simulink model "testemplanner_cs_old"  (R2020a)
settings: Solver=ode5  StartTime=0.0  StopTime=30  FixedStep=1/1000  RelTol=1e-3
PreLoadFcn:
  | mbxruntime.callbacks.PreLoadFcn(bdroot);
PostLoadFcn:
  | mbxruntime.callbacks.PostLoadFcn(bdroot);
InitFcn:
  | mbxruntime.callbacks.InitFcn(bdroot);
StartFcn:
  | mbxruntime.callbacks.StartFcn(bdroot);
StopFcn:
  | mbxruntime.callbacks.StopFcn(bdroot);
model workspace (MAT data in the model file):
  mbox_table : object (value not decoded)
  model_closed = 0
  sim_status = 0
values from neighbouring files (symbols this model uses):
  c_factor = 43.75    [emplanner_init.m]
  cf = -175016    [emplanner_init.m]
  cr = -130634    [emplanner_init.m]
  global_path_x = [-12.787 -11.7876177449 -10.7894946344 -9.79264775065 -8.79708287721 -7.80280164192 -6.80980414431 -5.81808992236 -4.82765830817 -3.83850855887 -2.85063990477 -1.86405156707 ... (3001 elements, 3001x1)]    [global_path.mat]
  global_path_y = [5.7602 5.7602 5.7602 5.7602 5.7602 5.7602 5.7602 5.7602 5.7602 5.7602 5.7602 5.7602 ... (3001 elements, 3001x1)]    [global_path.mat]
  KD_PID_distance = 0.0    (= 0)    [emplanner_init.m]
  KD_PID_speed = 0    [emplanner_init.m]
  KI_PID_distance = 0.0    (= 0)    [emplanner_init.m]
  KI_PID_speed = 0    [emplanner_init.m]
  KP_PID_distance = 0.5    [emplanner_init.m]
  KP_PID_speed = 1.8    [emplanner_init.m]
  la = 1.265    [emplanner_init.m]
  lb = 2.947-1.265    (= 1.682)    [emplanner_init.m]
  LQR_K1 = k(:,1)'    [emplanner_init.m]
  LQR_K2 = k(:,2)'    [emplanner_init.m]
  LQR_K3 = k(:,3)'    [emplanner_init.m]
  LQR_K4 = k(:,4)'    [emplanner_init.m]
  m = 2020    [emplanner_init.m]
  rack_displacement = [-39.14 , -37.2 , -35.29 , -33.43 , -31.6 , -29.81 , -28.06 , -26.34 , -24.66 ,      -23.01 , -21.38 , -19.79 , -18.23 , -16.69 , -15.18 , -13.7 , -12.23 , -10.8 , -9.38 , -7.98 ,     -6.61 , -5.25 , -3.91 , -2.59 , -1.29 , 0 , 1.27 , 2.54 , 3.78 , 5.02 , 6.24 , 7.46 , 8.66 ,      9.86 , 11.05 , 12.24 , 13.41 , 14.59 , 15.76 , 16.92 , 18.09 , 19.25 , 20.42 , 21.59 , 22.76 ,      23.93 , 25.11 , 26 ...(+26 chars)    [emplanner_init.m]
  right_wheel_ground = [-70 ,-67.2 , -64.4 , -61.6 , -58.8 , -56 , -53.2 , -50.4 , -47.6 , -44.8 , -42 ,      -39.2 , -36.4 , -33.6 , -30.8 , -28 , -25.2 , -22.4 , -19.6 , -16.8 , -14 , -11.2 , -8.4 , -5.6 ,      -2.8 , 0 , 2.8 , 5.6 , 8.4 , 11.2 , 14 , 16.8 , 19.6 , 22.4 , 25.2 , 28 , 30.8 , 33.6 , 36.4 ,      39.2 , 42 , 44.8 , 47.6 , 50.4 , 53.2 , 56 , 58.8 , 61.6 , 64.4 , 67.2 , 70 ]    [emplanner_init.m]
  vx_break_point = zeros(1,5000)    [emplanner_init.m]
undefined symbols (not defined in the file or in its folder): aubr, DiscIntNeverNeededParam, tablebr, vubr, warningInitialVelocity, x0
libraries: PreScanSimulinkLibrary x39, simulink x19, simulink_extras x11, Solver_SF x1
(part 12 of 17)

== matlab function testemplanner_cs_old/Audi_A8_Sedan_1/decision&planning module/EM Planner/path decision task1/path decision with dynamic planning(dp) ==
  data: obs_s_set input; dp_path_s output; obs_l_set input; plan_start_s input; plan_start_l input; plan_start_dl input; plan_start_dll input; w_cost_collision input; w_cost_smooth_dl input; w_cost_smooth_ddl input; w_cost_smooth_dddl input; w_cost_ref input; row input; col input; sample_s input; sample_l input; dp_path_l output
function [dp_path_s,dp_path_l] = fcn(obs_s_set,obs_l_set,plan_start_s,plan_start_l,plan_start_dl,...
    plan_start_dll,w_cost_collision,w_cost_smooth_dl,w_cost_smooth_ddl,w_cost_smooth_dddl,w_cost_ref,row,col,sample_s,sample_l)
%该函数为路径决策算法动态规划的主函数
% 输入：obs s l set 筛选后的障碍物sl信息
%       plan_start s l dl ddl 规划起点信息
%       w_cost_obs,w_cost_smooth_dl,w_cost_smooth_ddl,w_cost_smooth_dddl,w_cost_ref动态规划代价权重
%       row col 动态规划采样点的行数和列数(row必须是奇数，col必须是6)
%       sample_s,sample_l 采样的s l 长度
% 输出：dp_path_l,dp_path_s 动态规划的路径sl,此路径不包含规划起点  

%动态规划最优的数据结构是结构体矩阵，但是simulink不支持结构体矩阵，所以动态规划算法写的相对难以理解

%声明二维矩阵变量node_cost，node_cost(i,j)表示从起点出发，到行i列j节点的最小代价为node_cost(i,j)
node_cost = ones(row,col)*inf;%初始化为无穷大

%声明二维矩阵变量pre_node_index pre_node_index(i,j)表示从起点到行i列j的节点的最优路径中前一个节点的行号为
%pre_node_index(i,j)
%例：比如一条最优路径为 起点 -> node(1,1) -> node(2,2) -> node(3,3)
%则pre_node_index(3,3) = 2 (最优路径的前一个节点是node(2,2) 取它的行号）
%  pre_node_index(2,2) = 1 (最优路径的前一个节点是node(1,1) 取它的行号）
%  pre_node_index(1,1) = 0 (起点的行号默认是0)

% 其实pre_node_index就是当找到最小代价的路径后从终点到起点反向选择出最优路径的
%如果用结构体矩阵完全没有必要弄得这么麻烦，但是simulink不支持
pre_node_index = zeros(row,col);%初始化，所有节点的上个最优节点的行号都是0，也就是起点

%先计算从起点到第一列的cost
for i = 1:row
    node_cost(i,1) = CalcStartCost(plan_start_s,plan_start_l,plan_start_dl,...
    plan_start_dll,i,sample_s,sample_l,w_cost_collision,w_cost_smooth_dl,...
    w_cost_smooth_ddl,w_cost_smooth_dddl,w_cost_ref,obs_s_set,obs_l_set,row);
end
% 动态规划主函数，从第二列开始
for j = 2:col
    for i = 1:row
        %计算当前node(i,j)的s l
        cur_node_s = plan_start_s + j * sample_s;
        cur_node_l = ((row + 1)/2 - i) * sample_l;
        %遍历前一列的节点
        for k = 1:row
            %计算前一列节点的s l
            pre_node_s = plan_start_s + (j - 1) * sample_s;
            pre_node_l = ((row + 1)/2 - k) * sample_l;
            cost_neighbour = CalcNeighbourCost(pre_node_s,pre_node_l,cur_node_s,cur_node_l,w_cost_collision,...
    w_cost_smooth_dl,w_cost_smooth_ddl,w_cost_smooth_dddl,w_cost_ref,obs_s_set,obs_l_set);
            %起点到上一个节点的最小代价为node_cost(k,j-1)
            pre_min_cost = node_cost(k,j-1);
            %起点到node_cost(i,j)的最小代价 为node_cost(k,j-1)
            %再加上node(k,j-1)到node(i,j)的代价 (k = 1,2,3,4...row) 中最小的
            cost_temp = pre_min_cost + cost_neighbour;
            if cost_temp < node_cost(i,j)
                node_cost(i,j) = cost_temp;
                %把最优路径上一列节点的行号记录下来
                pre_node_index(i,j) = k;
            end
        end      
    end
end
%找到node_cost最后一列中，cost最小的，记代价最小的行号为index
index = 0;
min_cost = inf;
for i = 1:row
    if node_cost(i,end) < min_cost
        min_cost = node_cost(i,end);
        index = i;
    end
end
%动态规划最优路径初始化
dp_node_list_row = zeros(col,1);
%从后往前逆推
cur_index = index;
for i = 1:col
    %记录cur_index前面节点的行号
    pre_index = pre_node_index(cur_index,end - i + 1);
    %把cur_index放到dp_node_list_row对应的位置
    dp_node_list_row(col - i + 1) = cur_index;
    %再把pre_index 赋给 cur_index 进行下一步递推
    cur_index = pre_index;
end
% 输出初始化，由于事先不知道横纵向的采样列数，因此需要做缓冲
dp_path_s = ones(15,1)*-1;
dp_path_l = ones(15,1)*-1;
for i = 1:col
    dp_path_s(i) = plan_start_s + i * sample_s;
    dp_path_l(i) = ((row + 1) / 2 - dp_node_list_row(i)) * sample_l;
end








end
function cost = CalcNeighbourCost(pre_node_s,pre_node_l,cur_node_s,cur_node_l,w_cost_collision,...
    w_cost_smooth_dl,w_cost_smooth_ddl,w_cost_smooth_dddl,w_cost_ref,obs_s_set,obs_l_set)
% 该函数将计算相邻两个节点之间的cost
  
    start_l = pre_node_l;
    start_dl = 0;
    start_ddl = 0;
    end_l = cur_node_l;
    end_dl = 0;
    end_ddl = 0;
    start_s = pre_node_s;
    end_s = cur_node_s;
    coeff = CalcQuinticCoeffient(start_l,start_dl,start_ddl,end_l,end_dl,end_ddl,start_s,end_s);
    a0 = coeff(1);
    a1 = coeff(2);
    a2 = coeff(3);
    a3 = coeff(4);
    a4 = coeff(5);
    a5 = coeff(6);
    % 取10个点计算cost
    ds = zeros(10,1);
    l = zeros(10,1);
    dl = zeros(10,1);
    ddl = zeros(10,1);
    dddl = zeros(10,1);
    for i = 1:10
        ds(i) = start_s + (i-1)*(end_s - start_s)/10;
    end
    l = a0 * ones(10,1) + a1 * ds + a2 * ds.^2 + a3 * ds.^3 + a4 * ds.^4 + a5 * ds.^5;
    dl = a1 * ones(10,1) + 2 * a2 * ds + 3 * a3 * ds.^2 + 4 * a4 * ds.^3 + 5 * a5 * ds.^4;
    ddl = 2 * a2 * ones(10,1) + 6 * a3 * ds + 12 * a4 * ds.^2 + 20 * a5 * ds.^3;
    dddl = 6 * ones(10,1) * a3 + 24 * a4 * ds + 60 * a5 * ds.^2;
    cost_smooth = w_cost_smooth_dl * (dl' * dl) + w_cost_smooth_ddl * (ddl' * ddl) + w_cost_smooth_dddl * (dddl' * dddl);
    for i = 1:length(ddl)
        if abs(ddl(i))> 0.5 || abs(atan(dl(i))) > 0.4*pi
            cost_smooth = cost_smooth + 1e7;
            break;
        end
    end
    cost_ref = w_cost_ref * (l' * l);
    cost_collision = 0;
    for i = 1:length(obs_s_set)
        if isnan(obs_s_set(i))
            break;
        end
        dlon = ones(10,1) * obs_s_set(i) - ds;
        dlat = ones(10,1) * obs_l_set(i) - l;
        %这里做了非常简化的质点模型，认为障碍物就是一个点
        square_d = dlon.^2 + dlat.^2;
        cost_collision_once = CalcObsCost(w_cost_collision,square_d);
        cost_collision = cost_collision + cost_collision_once;
        % 判断障碍物的左右
        v1 = [ds(end);l(end)] - [ds(1);l(1)];
        v2 = [obs_s_set(i);obs_l_set(i)] - [ds(1);l(1)];
        flag = v1(1)*v2(2) - v1(2)*v2(1);
        if flag < 0 && cost_collision > 0
            cost_collision = cost_collision - 1000;
        end
    end
    
    cost = cost_collision + cost_smooth + cost_ref;


end


function cost = CalcStartCost(begin_s,begin_l,begin_dl,begin_ddl,cur_node_row,sample_s,sample_l,w_cost_collision,...
    w_cost_smooth_dl,w_cost_smooth_ddl,w_cost_smooth_dddl,w_cost_ref,obs_s_set,obs_l_set,row)
    %该函数将计算起点到第一层的cost
    start_l = begin_l;
    start_dl = begin_dl;
    start_ddl = begin_ddl;
    %  . . .
    %  . . . row = 3 中间的行号 = (row + 1) /2 = 2
    %  . . .
    end_l = ((row + 1)/2 - cur_node_row)*sample_l;
    end_dl = 0;
    end_ddl = 0;
    start_s = begin_s;
    end_s = begin_s + sample_s;
    coeff = CalcQuinticCoeffient(start_l,start_dl,start_ddl,end_l,end_dl,end_ddl,start_s,end_s);
    a0 = coeff(1);
    a1 = coeff(2);
    a2 = coeff(3);
    a3 = coeff(4);
    a4 = coeff(5);
    a5 = coeff(6);
    % 取10个点计算cost
    ds = zeros(10,1);
    l = zeros(10,1);
    dl = zeros(10,1);
    ddl = zeros(10,1);
    dddl = zeros(10,1);
    for i = 1:10
        ds(i) = start_s + (i-1)*sample_s/10;
    end
    l = a0 * ones(10,1) + a1 * ds + a2 * ds.^2 + a3 * ds.^3 + a4 * ds.^4 + a5 * ds.^5;
    dl = a1 * ones(10,1) + 2 * a2 * ds + 3 * a3 * ds.^2 + 4 * a4 * ds.^3 + 5 * a5 * ds.^4;
    ddl = 2 * a2 * ones(10,1) + 6 * a3 * ds + 12 * a4 * ds.^2 + 20 * a5 * ds.^3;
    dddl = 6 * ones(10,1) * a3 + 24 * a4 * ds + 60 * a5 * ds.^2;
    cost_smooth = w_cost_smooth_dl * (dl' * dl) + w_cost_smooth_ddl * (ddl' * ddl) + w_cost_smooth_dddl * (dddl' * dddl);
    for i = 1:length(dl)
        if abs(ddl(i))> 0.5 || abs(atan(dl(i))) > 0.4*pi
            cost_smooth = cost_smooth + 1e7;
            break;
        end
    end
    cost_ref = w_cost_ref * (l' * l);
    cost_collision = 0;
    for i = 1:length(obs_s_set)
        if isnan(obs_s_set(i))
            break;
        end
        dlon = ones(10,1) * obs_s_set(i) - ds;
        dlat = ones(10,1) * obs_l_set(i) - l;
        %这里做了非常简化的质点模型，认为障碍物就是一个点
        square_d = dlon.^2 + dlat.^2;
        cost_collision_once = CalcObsCost(w_cost_collision,square_d);
        cost_collision = cost_collision + cost_collision_once;
        % 判断障碍物的左右
        v1 = [ds(end);l(end)] - [ds(1);l(1)];
        v2 = [obs_s_set(i);obs_l_set(i)] - [ds(1);l(1)];
        flag = v1(1)*v2(2) - v1(2)*v2(1);
        if flag < 0 && cost_collision > 0
            cost_collision = cost_collision - 1000;
        end
    end
    
    cost = cost_collision + cost_smooth + cost_ref;
        
end

function obs_cost = CalcObsCost(w_cost_collision,square_d)
%该函数将计算障碍物的距离代价
% 暂定超过4米的cost为0 在4到3米的cost为1000/squard_d,在小于3米的cost为w_cost_collision
%   cost = 0;
%   for i = 1:length(square_d)
%       if (square_d(i) < 16 && square_d(i) > 9) 
%           cost = cost + 500/square_d(i);
%       elseif (square_d(i) <= 9)
%           cost = cost + w_cost_collision;
%       end
%   end
%   obs_cost = cost;
min_d = inf;
for i = 1:length(square_d)
    min_d = min(min_d,square_d(i));
end
    obs_cost = w_cost_collision * 10^(-min_d/3);
end

function coeff = CalcQuinticCoeffient(start_l,start_dl,start_ddl,end_l,end_dl,end_ddl,start_s,end_s)
    % l = a0 + a1*s + a2*s^2 + a3*s^3 + a4*s^4 + a5*s^5
    % l' = a1 + 2 * a2 * s + 3 * a3 * s^2 + 4 * a4 * s^3 + 5 * a5 * s^4
    % l'' = 2 * a2 + 6 * a3 * s + 12 * a4 * s^2 + 20 * a5 * s^3
    start_s2 = start_s * start_s;
    start_s3 = start_s2 * start_s;
    start_s4 = start_s3 * start_s;
    start_s5 = start_s4 * start_s;
    end_s2 = end_s * end_s;
    end_s3 = end_s2 * end_s;
    end_s4 = end_s3 * end_s;
    end_s5 = end_s4 * end_s;
    A = [1,start_s, start_s2,     start_s3,     start_s4,      start_s5;
         0 1,       2 * start_s,  3 * start_s2, 4 * start_s3,  5 * start_s4;
         0 0,       2,            6 * start_s,  12 * start_s2, 20 * start_s3;
         1,end_s, end_s2,     end_s3,     end_s4,      end_s5;
         0,1,     2 * end_s,  3 * end_s2, 4 * end_s3,  5 * end_s4;
         0,0,     2,          6 * end_s,  12 * end_s2, 20 * end_s3;];
    B = [start_l;
         start_dl;
         start_ddl;
         end_l;
         end_dl;
         end_ddl;];
     coeff = A \ B;
    
end

== matlab function testemplanner_cs_old/Audi_A8_Sedan_1/decision&planning module/referenceline provider/MATLAB Function4 ==
  data: referenceline_x_init input; referenceline_x output; referenceline_y_init input; w_cost_smooth input; w_cost_length input; w_cost_ref input; x_lb input; x_ub input; y_lb input; y_ub input; referenceline_y output
function [referenceline_x,referenceline_y] = ...
    fcn(referenceline_x_init,referenceline_y_init,w_cost_smooth,w_cost_length,w_cost_ref,x_lb,x_ub,y_lb,y_ub)
%该函数用于平滑referenceline
%使用二次规划
% 0.5x'Hx + f'x = min
% lb < x < ub
% 输入： referenceline_x_init,referenceline_y_init未平滑的参考线
%       w_cost_smooth,w_cost_length,w_cost_ref 平滑代价、紧凑代价、几何相似代价权重系数
%       x_lb,x_ub,y_lb,y_ub 允许x，y变化的上下界
%输出：referenceline_x,referenceline_y 平滑后的参考线

% 在这里为了简化，不使用参考线拼接算法
% 计算量问题通过调度解决，规划周期为100ms，只要在100ms内计算完就可以
% 如果到最后计算速度成问题再优化，目前暂时不适用拼接

% simulink无法直接使用自带的二次规划函数，需要从外部引入

coder.extrinsic("quadprog")
% 二次规划形式 （详见第二章第二节上）
% H1 = w_cost_smooth*(A1'*A1) + w_cost_length*(A2'*A2) + w_cost_ref*(A3'*A3)
% f = -2 * w_cost_ref * referenceline_init
% x'H1x + f'x = 0.5 * x'(2H1) * x + f'x
% A1 = [1  0 -2  0  1  0
%       0  1  0 -2  0  1
%             1  0 -2  0  1  0
%             0  1  0 -2  0  1
%                   ...............
% A2 = [1  0 -1  0
%      0  1  0 -1
%            1  0 -1  0
%            0  1  0 -1
%                  ...........
% A3 为单位矩阵
%设置求解矩阵规模，因为参考线初始点一共181个，每个点有两个坐标，所以求解矩阵规模是362个
n = 181;
%referenceline初始化
referenceline_x = zeros(n,1);
referenceline_y = zeros(n,1);

A1 = zeros(2 * n - 4, 2 * n);
A2 = zeros(2 * n - 2, 2 * n);
A3 = eye(2 * n, 2 * n);
f = zeros(2 * n, 1);
lb = zeros(2 * n, 1);
ub = zeros(2 * n, 1);
persistent is_first_run;
persistent pre_result_x;
persistent pre_result_y;
persistent pre_referenceline_x_init;
persistent pre_referenceline_y_init;

if isempty(is_first_run)
    is_first_run = 0;
    for i = 1 : n
        f(2 * i - 1) = referenceline_x_init(i);
        f(2 * i) = referenceline_y_init(i);
        lb(2 * i - 1) = f(2 * i - 1) + x_lb;
        ub(2 * i - 1) = f(2 * i - 1) + x_ub;
        lb(2 * i) = f(2 * i) + y_lb;
        ub(2 * i) = f(2 * i) + y_ub;
    end

    for j = 1 : 2 : 2 * n - 5   %A1维度2n-4 * 2n
        A1(j , j) = 1;
        A1(j , j + 2) = -2;
        A1(j , j + 4) = 1;
        A1(j + 1, j + 1) = 1;
        A1(j + 1, j + 3) = -2;
        A1(j + 1, j + 5) = 1;
    end

    for k = 1 : 2: 2 * n - 3
        A2(k, k) = 1;
        A2(k, k + 2) = -1;
        A2(k + 1, k + 1) = 1;
        A2(k + 1, k + 3) = -1;
    end

    H1 = w_cost_smooth * (A1'*A1) + w_cost_length * (A2'*A2) + w_cost_ref * (A3);
    H = 2 * H1;
    %用 referenceline 的初值作为二次规划的迭代起点
    X0 = f;
    f = -2 * w_cost_ref * f;
    %二次规划求解
    X = quadprog(H,f,[],[],[],[],lb,ub,X0);
    %将结果输出到referenceline中
    for i = 1 : n
       referenceline_x(i) = X(2 * i - 1);
       referenceline_y(i) = X(2 * i);
    end
    pre_result_x = referenceline_x;
    pre_result_y = referenceline_y;
    pre_referenceline_x_init = referenceline_x_init;
    pre_referenceline_y_init = referenceline_y_init;
else
    %起点相同，可以认为本周期和上周期的referenceline_init 一模一样，就直接复用上个周期的结果
    if pre_referenceline_x_init(1) == referenceline_x_init(1) && ...
            pre_referenceline_y_init(1) == referenceline_y_init(1)
        referenceline_x = pre_result_x;
        referenceline_y = pre_result_y;
    else
        %起点不同。重复第一次运行的逻辑
        for i = 1 : n
            f(2 * i - 1) = referenceline_x_init(i);
            f(2 * i) = referenceline_y_init(i);
            lb(2 * i - 1) = f(2 * i - 1) + x_lb;
            ub(2 * i - 1) = f(2 * i - 1) + x_ub;
            lb(2 * i) = f(2 * i) + y_lb;
            ub(2 * i) = f(2 * i) + y_ub;
        end

        for j = 1 : 2: 2 * n - 5
            A1(i , i) = 1;
            A1(i , i + 2) = -2;
            A1(i , i + 4) = 1;
            A1(i + 1, i + 1) = 1;
            A1(i + 1, i + 3) = -2;
            A1(i + 1, i + 5) = 1;
        end

        for k = 1 : 2: 2 * n - 3
            A2(i, i) = 1;
            A2(i, i + 2) = -1;
            A2(i + 1, i + 1) = 1;
            A2(i + 1, i + 3) = -1;
        end

        H1 = w_cost_smooth * (A1'*A1) + w_cost_length * (A2'*A2) + w_cost_ref * A3;
        H = 2 * H1;
        %用 referenceline 的初值作为二次规划的迭代起点
        X0 = f;
        f = -2 * w_cost_ref * f;
        %二次规划求解
        X = quadprog(H,f,[],[],[],[],lb,ub,X0);
        %将结果输出到referenceline中
        for i = 1 : n
            referenceline_x(i) = X(2 * i - 1);
            referenceline_y(i) = X(2 * i);
        end
        pre_result_x = referenceline_x;
        pre_result_y = referenceline_y;
        pre_referenceline_x_init = referenceline_x_init;
        pre_referenceline_y_init = referenceline_y_init;        
    end
end

== matlab function testemplanner_cs_old/Audi_A8_Sedan_1/decision&planning module/EM Planner/path planning task1/MATLAB Function ==
  data: qp_path_s input; qp_path_s_final output; qp_path_l input; qp_path_dl input; qp_path_ddl input; qp_path_l_final output; qp_path_dl_final output; qp_path_ddl_final output
function [qp_path_s_final,qp_path_l_final, qp_path_dl_final,qp_path_ddl_final] = fcn(qp_path_s,qp_path_l,qp_path_dl,qp_path_ddl)
% 该函数将增密qp_path
n_init = 20;
% 增密的点的个数
n = 501;
% 输出初始化
qp_path_s_final = zeros(n,1);
qp_path_l_final = zeros(n,1);
qp_path_dl_final = zeros(n,1);
qp_path_ddl_final = zeros(n,1);
ds = (qp_path_s(end) - qp_path_s(1))/(n-1);
index = 1;
for i = 1:n
    x = qp_path_s(1) + (i-1) * ds;
    qp_path_s_final(i) = x;
    while x >= qp_path_s(index)
        index = index + 1;
        if index == n_init
            break;
        end
    end
    % while 循环退出的条件是x<qp_path_s(index)，所以x对应的前一个s的编号是index-1 后一个编号是index
    pre = index - 1;
    cur = index;
    % 计算前一个点的l l' l'' ds 和后一个点的 l''
    delta_s = x - qp_path_s(pre);
    l_pre = qp_path_l(pre);
    dl_pre = qp_path_dl(pre);
    ddl_pre = qp_path_ddl(pre);
    ddl_cur = qp_path_ddl(cur);
    % 分段加加速度优化 
    qp_path_l_final(i) = l_pre + dl_pre * delta_s + (1/3)* ddl_pre * delta_s^2 + (1/6) * ddl_cur * delta_s^2;
    qp_path_dl_final(i) = dl_pre + 0.5 * ddl_pre * delta_s + 0.5 * ddl_cur * delta_s;
    qp_path_ddl_final(i) = ddl_pre + (ddl_cur - ddl_pre) * delta_s/(qp_path_s(cur) - qp_path_s(pre));
    %  因为此时x的后一个编号是index 必有x < qp_path_s(index),在下一个循环中x = x + ds 也未必大于
    %  qp_path_s(index)，这样就进入不了while循环，所以index 要回退一位
    index = index - 1;   
end

== matlab function testemplanner_cs_old/Audi_A8_Sedan_1/decision&planning module/EM Planner/path planning task1/generate convex space ==
  data: dp_path_s input; l_min output; dp_path_l input; static_obs_s_set input; static_obs_l_set input; static_obs_length input; static_obs_width input; l_max output
function [l_min,l_max] = fcn(dp_path_s,dp_path_l,static_obs_s_set,static_obs_l_set,static_obs_length,static_obs_width)
    % 该函数将输出每个离散的dp_path_s所对应的l的边界lmin lmax (本质上是质点的凸空间)
    % 输入 动态规划曲线 dp_path_s,dp_path_l
    %      障碍物中心的s l 坐标 static_obs_s,static_obs_l
    %      障碍物的长宽 static_obs_length,static_obs_width 
    % 输出 l_min lmax l 的上下界

    % 输出初始化
    l_min = ones(60,1) * -8;
    l_max = ones(60,1) * 8;
    % 对每个障碍物做遍历
    for i = 1:length(static_obs_s_set)
        if isnan(static_obs_s_set(i))
            break;
        end
        % 计算障碍物的头部和尾部的s
        obs_s_min = static_obs_s_set(i) - static_obs_length/2;
        obs_s_max = static_obs_s_set(i) + static_obs_length/2;
        % 找到dp_path_s 中，与s_head s_end最近的s的编号
        start_index = FindNearIndex(dp_path_s,obs_s_min);
        end_index = FindNearIndex(dp_path_s,obs_s_max);
        path_l = (dp_path_l(start_index) + dp_path_l(end_index))/2;
        if start_index == 1 && end_index == 1
            continue;
        end
        if path_l > static_obs_l_set(i)
            % 意味着决策为向左绕过障碍物
            for j = start_index:end_index
                % l_min(j) 为所有决策为向左绕过障碍物的l边界的最大值
                l_min(j) = max(l_min(j) , static_obs_l_set(i) + static_obs_width/2);
            end
        else
            % 意味着决策为向右绕过障碍物
            for j = start_index:end_index
                % l_max(j) 为所有决策为向右绕过障碍物的l边界的最小值
                l_max(j) = min(l_max(j) , static_obs_l_set(i) - static_obs_width/2);
            end
        end       
    end
end

function y = FindNearIndex(dp_path_s,obs_s)
    % 该函数将找到dp_path_s的所有点中，距离obs_s最近的点的编号
    % 这里要注意obs_s 是在完整的reference line上投影所得到的坐标，所以obs_s可能是负值，也可能会超过dp_path_s最远的长度
    if dp_path_s(1) >= obs_s
        %障碍物在后面
        y = 1;
        return;
    elseif dp_path_s(end) <= obs_s
        y = 60;
        return;
    else
        index = 1;
        while dp_path_s(index) < obs_s
            index = index + 1;
        end
        % 循环退出的条件是dp_path_s(index) >= obs_s 判断一下index 和 index-1哪个离的近
        if dp_path_s(index) - obs_s > obs_s - dp_path_s(index - 1)
            y = index - 1;
        else
            y = index;
        end
    end
end

== matlab function testemplanner_cs_old/Audi_A8_Sedan_1/decision&planning module/EM Planner/path planning task1/path planning with quadratic programming (qp) ==
  data: qp_path_s output; l_min input; qp_path_l output; l_max input; w_cost_l input; w_cost_dl input; w_cost_ddl input; w_cost_dddl input; w_cost_centre input; w_cost_end_l input; w_cost_end_dl input; w_cost_end_ddl input; host_d1 input; host_d2 input; host_w input; plan_start_s input; plan_start_l input; plan_start_dl input; plan_start_ddl input; qp_path_dl output; qp_path_ddl output; delta_dl_max input; delta_ddl_max input
function [qp_path_s,qp_path_l,qp_path_dl,qp_path_ddl] = ...
fcn(l_min,l_max,w_cost_l,w_cost_dl,w_cost_ddl,w_cost_dddl,w_cost_centre,w_cost_end_l,w_cost_end_dl,w_cost_end_ddl,...
    host_d1,host_d2,host_w,...
    plan_start_s,plan_start_l,plan_start_dl,plan_start_ddl,...
    delta_dl_max,delta_ddl_max)
% 路径二次规划
% 0.5*x'Hx + f'*x = min
% subject to A*x <= b
%            Aeq*x = beq
%            lb <= x <= ub;
% 输入：l_min l_max 点的凸空间
%       w_cost_l 参考线代价
%       w_cost_dl ddl dddl 光滑性代价
%       w_cost_centre 凸空间中央代价
%       w_cost_end_l dl dd1 终点的状态代价 (希望path的终点状态为(0,0,0))
%       host_d1,d2 host质心到前后轴的距离
%       host_w host的宽度
%       plan_start_l,dl,ddl 规划起点
% 输出 qp_path_l dl ddl 二次规划输出的曲线
coder.extrinsic("quadprog");
% 待优化的变量的数量
n = 20;

% 输出初始化
qp_path_l = zeros(n,1);
qp_path_dl = zeros(n,1);
qp_path_ddl = zeros(n,1);
qp_path_s = zeros(n,1);

% H_L H_DL H_DDL H_DDDL Aeq beq A b 初始化
H_L = zeros(3*n, 3*n);
H_DL = zeros(3*n, 3*n);
H_DDL = zeros(3*n, 3*n);
H_DDDL = zeros(n-1, 3*n);
H_CENTRE = zeros(3*n, 3*n);
H_L_END = zeros(3*n, 3*n);
H_DL_END = zeros(3*n, 3*n);
H_DDL_END = zeros(3*n, 3*n);
Aeq = zeros(2*n-2, 3*n);
beq = zeros(2*n-2, 1);
A = zeros(8*n, 3*n);
b = zeros(8*n, 1);
% 更新：加入 dl(i+1) - dl(i) ddl(i+1) - ddl(i) 的约束
A_dl_minus = zeros(n - 1,3*n);
b_dl_minus = zeros(n - 1,1);
A_ddl_minus = zeros(n - 1,3*n);
b_ddl_minus = zeros(n - 1,1);
for i = 1:n-1
    row = i;
    col = 3*i - 2;
    A_dl_minus(row,col:col+5) = [0 -1 0 0 1 0];
    b_dl_minus(row) = delta_dl_max;
    A_ddl_minus(row,col:col+5) = [0 0 -1 0 0 1];
    b_ddl_minus(row) = delta_ddl_max;
end
% -max < a*x < max => ax < max && -ax < -(-max)
A_minus = [A_dl_minus;
          -A_dl_minus;
           A_ddl_minus;
          -A_ddl_minus];
b_minus = [b_dl_minus;
           b_dl_minus;
          b_ddl_minus;
          b_ddl_minus]; 

%  期望的终点状态
end_l_desire = 0;
end_dl_desire = 0;
end_ddl_desire = 0;

% Aeq_sub
ds = 3;%纵向间隔
for i = 1:n
    qp_path_s(i) = plan_start_s + (i-1)*ds;
end

Aeq_sub = [1 ds ds^2/3 -1 0 ds^2/6;
           0 1  ds/2   0 -1 ds/2];
% A_sub;
d1 = host_d1;
d2 = host_d2;
w = host_w;
A_sub = [1  d1 0;
         1  d1 0;
         1 -d2 0;
         1 -d2 0;
        -1 -d1 0;
        -1 -d1 0;
        -1  d2 0;
        -1  d2 0];
% 生成Aeq
for i = 1:n-1
    % 计算分块矩阵左上角的行和列
    row = 2*i - 1;
    col = 3*i - 2;
    Aeq(row:row + 1,col:col + 5) = Aeq_sub;
end
% 生成A
for i = 2:n
    row = 8*i - 7;
    col = 3*i - 2;
    A(row:row + 7,col:col + 2) = A_sub;
end

% 视频里用的找(s(i) - d2,s(i) + d1)的方法过于保守，在这里舍弃掉
% 只要找到四个角点所对应的l_min l_max 即可
% 。。。。。。。。。。。。。。
%    [    .   ]<- 
%    [        ]
% 。。。。。。。。。。。。。
front_index = ceil(d1/ds);
back_index = ceil(d2/ds); % ceil向上取整 ceil(3) = 3 ceil(3.1) = 4
% 生成b
for i = 2:n
    % 左前 右前的index = min(i + front_index,60)
    % 左后 右后的index = max(i - back_index,1)
    % l_min l_max 都是60个点
    index1 = min(3*i - 2 + front_index,n);
    index2 = max(3*i - 2 - back_index,1);
    b(8*i - 7:8*i,1) = [l_max(index1) - w/2;
                        l_max(index1) + w/2;
                        l_max(index2) - w/2;
                        l_max(index2) + w/2;
                       -l_min(index1) + w/2;
                       -l_min(index1) - w/2;
                       -l_min(index2) + w/2;
                       -l_min(index2) - w/2;];
end
%生成 lb ub 主要是对规划起点做约束
lb = ones(3*n,1)*-inf;
ub = ones(3*n,1)*inf;
lb(1) = plan_start_l;
lb(2) = plan_start_dl;
lb(3) = plan_start_ddl;
ub(1) = lb(1);
ub(2) = lb(2);
ub(3) = lb(3);
for i = 2:n
    lb(3*i - 1) = - 2; %约束 l'
    ub(3*i - 1) = 2;
    lb(3*i) = -0.1; %约束 l''
    ub(3*i) = 0.1;
end
% 生成H_L,H_DL,H_DDL,H_CENTRE
for i = 1:n
    H_L(3*i - 2,3*i - 2) = 1;
    H_DL(3*i - 1,3*i - 1) = 1;
    H_DDL(3*i, 3*i) = 1;
end
H_CENTRE = H_L;
% 生成H_DDDL;
H_dddl_sub = [0 0 1 0 0 -1];
for i = 1:n-1
    row = i;
    col = 3*i - 2;
    H_DDDL(row,col:col + 5) = H_dddl_sub;
end
% 生成H_L_END H_DL_END H_DDL_END
H_L_END(3*n - 2,3*n - 2) = 1;
H_DL_END(3*n - 1,3*n - 1) = 1;
H_DDL_END(3*n,3*n) = 1;
% 生成二次规划的H 因为ds ！= 1 所以 dddl = delta_ddl/ds;
H = w_cost_l * (H_L'*H_L) + w_cost_dl * (H_DL'*H_DL) + w_cost_ddl * (H_DDL'*H_DDL)...
   +w_cost_dddl * (H_DDDL'*H_DDDL)/ds + w_cost_centre * (H_CENTRE'*H_CENTRE) + w_cost_end_l * (H_L_END'*H_L_END)...
   +w_cost_end_dl * (H_DL_END'* H_DL_END) + w_cost_ddl * (H_DDL_END'*H_DDL_END);
H = 2 * H;
% 生成f
f = zeros(3*n,1);
 centre_line = 0.5 * (l_min + l_max); % 此时centre line 还是60个点
% centre_line = dp_path_l_final;
for i = 1:n
    f(3*i - 2) = -2 * centre_line(3*i - 2);
end
% 避免centreline权重过大影响轨迹平顺性
for i = 1:n
    if abs(f(i)) > 0.3
        f(i) = w_cost_centre * f(i);
    end
end
% 终点要接近end_l dl ddl desire
f(3*n - 2) = f(3*n - 2) -2 * end_l_desire * w_cost_end_l;
f(3*n - 1) = f(3*n - 1) -2 * end_dl_desire * w_cost_end_dl;
f(3*n) = f(3*n) -2 * end_ddl_desire * w_cost_end_ddl;

X = quadprog(H,f,A,b,Aeq,beq,lb,ub);

for i = 1:n
    qp_path_l(i) = X(3*i - 2);
    qp_path_dl(i) = X(3*i - 1);
    qp_path_ddl(i) = X(3*i);
end

end

== matlab function testemplanner_cs_old/Audi_A8_Sedan_1/decision&planning module/EM Planner/plot ==
  data: dp_s input; dp_l input; qp_s input; qp_l input; l_min input; l_max input; obs_s_set input; obs_l_set input; start_s input; start_l input; start_dl input
function  fcn(dp_s,dp_l,qp_s,qp_l,l_min,l_max,obs_s_set,obs_l_set,start_s,start_l,start_dl)
coder.extrinsic("plot","axis","figure","drawnow","cla","fill");

obs_length = 5;
obs_width = 2;
host_l = 6;
host_w = 1.63;
cla;
host_p1_l = start_l + sin(atan(start_dl)) * host_l /2 + host_w/2 * cos(atan(start_dl));
host_p1_s = start_s + cos(atan(start_dl)) * host_l /2 - host_w/2 * sin(atan(start_dl));
host_p2_l = start_l + sin(atan(start_dl)) * host_l /2 - host_w/2 * cos(atan(start_dl));
host_p2_s = start_s + cos(atan(start_dl)) * host_l /2 + host_w/2 * sin(atan(start_dl));
host_p3_l = start_l - sin(atan(start_dl)) * host_l /2 + host_w/2 * cos(atan(start_dl));
host_p3_s = start_s - cos(atan(start_dl)) * host_l /2 - host_w/2 * sin(atan(start_dl));
host_p4_l = start_l - sin(atan(start_dl)) * host_l /2 - host_w/2 * cos(atan(start_dl));
host_p4_s = start_s - cos(atan(start_dl)) * host_l /2 + host_w/2 * sin(atan(start_dl));
host_area_x = [host_p1_s;host_p2_s;host_p4_s;host_p3_s];
host_area_y = [host_p1_l;host_p2_l;host_p4_l;host_p3_l];
fill(host_area_x,host_area_y,[0 1 1]);
hold on
plot(dp_s,dp_l,'r');

plot(qp_s,qp_l,'b');
plot(dp_s,l_min,dp_s,l_max);
axis([-8 70 -10 10]);

for i = 1:length(obs_s_set)
    if isnan(obs_s_set(i))
        break;
    end
    obs_p1_s = obs_s_set(i) + obs_length/2;
    obs_p1_l = obs_l_set(i) + obs_width/2;
    obs_p2_s = obs_s_set(i) + obs_length/2;
    obs_p2_l = obs_l_set(i) - obs_width/2;
    obs_p3_s = obs_s_set(i) - obs_length/2;
    obs_p3_l = obs_l_set(i) + obs_width/2;
    obs_p4_s = obs_s_set(i) - obs_length/2;
    obs_p4_l = obs_l_set(i) - obs_width/2;
    obs_area_s = [obs_p1_s;obs_p2_s;obs_p4_s;obs_p3_s];
    obs_area_l = [obs_p1_l;obs_p2_l;obs_p4_l;obs_p3_l];
    fill(obs_area_s,obs_area_l,[0 0 0]);
end

== matlab function testemplanner_cs_old/Audi_A8_Sedan_1/decision&planning module/EM Planner/spee planning with quadratic programming (qp) ==
  data: plan_start_s_dot input; qp_s_init output; plan_start_s_dot2 input; dp_speed_s input; dp_speed_t input; s_lb input; s_ub input; s_dot_lb input; s_dot_ub input; qp_s_dot_init output; qp_s_dot2_init output; relative_time_init output; w_cost_s_dot2 input; w_cost_v_ref input; w_cost_jerk input; speed_reference input
function [qp_s_init,qp_s_dot_init,qp_s_dot2_init,relative_time_init] = fcn(plan_start_s_dot,...
    plan_start_s_dot2,dp_speed_s,dp_speed_t,s_lb,s_ub,s_dot_lb,s_dot_ub,w_cost_s_dot2,w_cost_v_ref,w_cost_jerk,speed_reference)
%速度二次规划
% 输入：规划起点plan_start_s_dot,plan_start_s_dot2
%       动态规划结果dp_speed_s,dp_speed_t
%       凸空间约束 s_lb,s_ub,s_dot_lb,s_dot_ub
%       加速度代价权重，推荐速度代价权重，jerk代价权重w_cost_s_dot2,w_cost_v_ref,w_cost_jerk
%       参考速度speed_reference
% 输出：速度曲线qp_s_init,qp_s_dot_init,qp_s_dot2_init,relative_time_init
coder.extrinsic("quadprog")
% 由于dp的结果未必是16，该算法将计算dp_speed_end到底是多少
dp_speed_end = 16;
for i = 1:length(dp_speed_s)
    
    if isnan(dp_speed_s(i))
        dp_speed_end = i - 1;
        break;
    end
end
% 由于dp_speed_end实际上是不确定的，但是输出要求必须是确定长度的值，因此
% 输出初始化选择dp_speed_end的最大值 + 规划起点作为输出初始化的规模
n = 17;

qp_s_init = ones(n,1) * nan;
qp_s_dot_init = ones(n,1) * nan;
qp_s_dot2_init = ones(n,1) * nan;
relative_time_init = ones(n,1) * nan;
s_end = dp_speed_s(dp_speed_end);
% 此时dp_speed_end表示真正有效的dp_speed_t的元素个数，取出dp_speed_t有效的最后一个元素作为规划的时间终点
% 记为recommend_T
recommend_T = dp_speed_t(dp_speed_end);
% qp的规模应该是dp的有效元素的个数 + 规划起点
qp_size = dp_speed_end + 1;
% 连续性约束矩阵初始化，这里的等式约束应该是 Aeq'*X == beq 有转置
Aeq = zeros(3*qp_size,2*qp_size - 2);
beq = zeros(2*qp_size - 2,1);
% 不等式约束初始化
lb = ones(3*qp_size,1);
ub = lb;
% 计算采样间隔时间dt
dt = recommend_T/dp_speed_end;
A_sub =[1,0;
        dt,1;
        (1/3)*dt^2,(1/2)*dt;
        -1,0;
        0,-1;
        (1/6)*dt^2,dt/2];
for i = 1:qp_size - 1
    Aeq(3*i-2:3*i+3,2*i-1:2*i) = A_sub;
end
% 这里初始化不允许倒车约束，也就是 s(i) - s(i+1) <= 0
A = zeros(qp_size-1,3*qp_size);
b = zeros(qp_size-1,1);
for i = 1:qp_size-1
    A(i,3*i - 2) = 1;
    A(i,3*i + 1) = -1;
end
% 由于生成的凸空间约束s_lb s_ub不带起点，所以lb(i) = s_lb(i-1) 以此类推
% 允许最小加速度为-6 最大加速度为4(基于车辆动力学)
for i = 2:qp_size
   lb(3*i - 2) = s_lb(i-1);
   lb(3*i - 1) = s_dot_lb(i-1);
   lb(3*i) = -6;
   ub(3*i - 2) = s_ub(i-1);
   ub(3*i - 1) = s_dot_ub(i-1);
   ub(3*i) = 4;
end
% 起点约束
lb(1) = 0;
lb(2) = plan_start_s_dot;
lb(3) = plan_start_s_dot2;
ub(1) = lb(1);
ub(2) = lb(2);
ub(3) = lb(3);
% 加速度代价 jerk代价 以及推荐速度代价
A_s_dot2 = zeros(3*qp_size,3*qp_size);
A_jerk = zeros(3*qp_size,qp_size - 1);
A_ref = zeros(3*qp_size,3*qp_size);

A4_sub =[0;0;1;0;0;-1];
for i = 1:qp_size
    A_s_dot2(3*i,3*i) = 1;
    A_ref(3*i-1,3*i-1) = 1;
end
for i = 1:qp_size - 1   
   A_jerk(3*i-2:3*i+3,i:i) = A4_sub;
end
% 生成H f
H = w_cost_s_dot2 * (A_s_dot2 * A_s_dot2') + w_cost_jerk * (A_jerk * A_jerk') + w_cost_v_ref * (A_ref * A_ref');
H = 2*H;
f = zeros(3*qp_size,1);
for i = 1:qp_size
    f(3*i-1) =  - 2 * w_cost_v_ref * speed_reference;
end
% 计算二次规划
X = quadprog(H,f,A,b,Aeq',beq,lb,ub);
% 将结果输出
for i = 1:qp_size
   qp_s_init(i) = X(3*i - 2);
   qp_s_dot_init(i) = X(3*i - 1);
   qp_s_dot2_init(i) = X(3*i);
   relative_time_init(i) = (i - 1)*dt;
end

== matlab function testemplanner_cs_old/Audi_A8_Sedan_1/decision&planning module/EM Planner/speed decision with dynamic planning(dp)1 ==
  data: obs_st_s_in_set input; dp_speed_s output; obs_st_s_out_set input; obs_st_t_in_set input; obs_st_t_out_set input; dp_speed_t output; reference_speed_unlimit input; w_cost_ref_speed input; w_cost_accel input; w_cost_obs input; plan_start_s_dot input
function [dp_speed_s,dp_speed_t] = fcn(obs_st_s_in_set,obs_st_s_out_set,obs_st_t_in_set,obs_st_t_out_set,reference_speed_unlimit...
    ,w_cost_ref_speed,w_cost_accel,w_cost_obs,plan_start_s_dot)
% 速度动态规划
% 时间从0到8开始规划，最多8秒
% s的范围从0开始到路径规划的path的总长度为止
% 为了减少算力 采用非均匀采样，s越小的越密，越大的越稀疏

s_list = [0:0.5:4.5,...
          5.5:1:14.5,...
          16:1.5:29.5,...
          32:2.5:54.5];
% t 采用均匀采样每 0.5s采样一个点
t_list = 0.5:0.5:8;
% 声明st代价矩阵，表示从起点开始到(i,j)点的最小代价为dp_st_cost(i,j)
% s 采样40个 t 采样 16个 一共是 40 * 16
dp_st_cost = ones(40,16) * inf; % 首先初始化为无穷大
% dp_st_s_dot，表示从起点开始到(i,j)点的最优路径的末速度
dp_st_s_dot = zeros(40,16);
% 需要一个矩阵保持最优路径的前一个节点方便回溯
% dp_st_node(i,j) 表示位置为(i,j)的节点中，最优的上一层节点的行号为dp_st_node(i,j)
dp_st_node = zeros(40,16);
% 计算从dp起点到第一列的cost
for i = 1:length(s_list)
    dp_st_cost(i,1) = CalcDpCost(0,0,i,1,obs_st_s_in_set,obs_st_s_out_set,obs_st_t_in_set,obs_st_t_out_set,...
    w_cost_ref_speed,reference_speed_unlimit,w_cost_accel,w_cost_obs,plan_start_s_dot,s_list,t_list,dp_st_s_dot);
    % 计算第一列所有节点的的s_dot，并存储到dp_st_s_dot中
    % 第一列的前一个节点只有起点，起点的s t 都是0
    [s_end,t_end] = CalcSTCoordinate(i,1,s_list,t_list);
    dp_st_s_dot(i,1) = s_end / t_end;
end
% 动态规划主程序
for i = 2:length(t_list)
    % i 为列循环
    for j = 1:length(s_list)
        % j 为行循环
        % 当前行为 j 列为 i
        cur_row = j;
        cur_col = i;
        % 遍历前一列
        for k = 1:length(s_list)
            pre_row = k;
            pre_col = i - 1;
            % 计算边的代价 其中起点为pre_row,pre_col 终点为cur_row cur_col
            cost_temp = CalcDpCost(pre_row,pre_col,cur_row,cur_col,obs_st_s_in_set,obs_st_s_out_set,...
                obs_st_t_in_set,obs_st_t_out_set,w_cost_ref_speed,reference_speed_unlimit,w_cost_accel,w_cost_obs,...
                plan_start_s_dot,s_list,t_list,dp_st_s_dot);
            if cost_temp + dp_st_cost(pre_row,pre_col) < dp_st_cost(cur_row,cur_col)
                dp_st_cost(cur_row,cur_col) = cost_temp + dp_st_cost(pre_row,pre_col);
                % 计算最优的s_dot
                [s_start,t_start] = CalcSTCoordinate(pre_row,pre_col,s_list,t_list);
                [s_end,t_end] = CalcSTCoordinate(cur_row,cur_col,s_list,t_list);
                dp_st_s_dot(cur_row,cur_col) = (s_end - s_start) / (t_end - t_start);
                % 将最短路径的前一个节点的行号记录下来
                dp_st_node(cur_row,cur_col) = pre_row;
            end      
        end
    end
end
% 输出初始化
dp_speed_s = ones(length(t_list),1) * nan;
dp_speed_t = dp_speed_s;
% 找到dp_node_cost 上边界和右边界代价最小的节点
min_cost = inf;
min_row = inf;
min_col = inf;
for i = 1:length(s_list)
    % 遍历右边界
    if dp_st_cost(i,length(t_list)) <= min_cost
        min_cost = dp_st_cost(i,length(t_list));
        min_row = i;
        min_col = length(t_list);
    end
end

for j = 1:length(t_list)
    % 遍历上边界
    if dp_st_cost(1,j) <= min_cost
        min_cost = dp_st_cost(1,j);
        min_row = 1;
        min_col = j;
    end
end
% 这里要注意，虽然我们在t上每0.5s采样一个时间，采了16个点，但是min_col 未必等于16
% 也就是说动态规划的最优解的时间未必是8秒
% 所以我们动态规划最后的输出s t 不一定是写满
% 先把终点的ST输出出来
[dp_speed_s(min_col),dp_speed_t(min_col)] = CalcSTCoordinate(min_row,min_col,s_list,t_list);
% 反向回溯
while min_col ~= 1
    pre_row = dp_st_node(min_row,min_col);
    pre_col = min_col - 1;
    [dp_speed_s(pre_col),dp_speed_t(pre_col)] = CalcSTCoordinate(pre_row,pre_col,s_list,t_list);
    min_row = pre_row;
    min_col = pre_col;
end


end

function cost = CalcDpCost(row_start,col_start,row_end,col_end,obs_st_s_in_set,obs_st_s_out_set,obs_st_t_in_set,obs_st_t_out_set,...
    w_cost_ref_speed,reference_speed,w_cost_accel,w_cost_obs,plan_start_s_dot,s_list,t_list,dp_st_s_dot)
    % 该函数将计算链接两个节点之间边的代价
    % 输入：边的起点的行列号row_start,col_start 边的终点行列号row_end,col_end
          % 障碍物st信息obs_st_s_in_set,obs_st_s_out_set,obs_st_t_in_set,obs_st_t_out_set
          % 推荐速度代价权重w_cost_ref_speed,加速度代价权重w_cost_accel,障碍物代价权重w_cost_obs
          % 推荐速度reference_speed
          % 拼接起点的速度plan_start_s_dot
          % s_list,t_list 采样距离
          % dp_st_s_dot 用于计算加速度
    % 首先计算终点的st坐标
    [s_end,t_end] = CalcSTCoordinate(row_end,col_end,s_list,t_list);
    % 规定起点的行列号为0 
    if row_start == 0
        % 边的起点为dp的起点
        s_start = 0;
        t_start = 0;
        s_dot_start = plan_start_s_dot;
    else
        % 边的起点不是dp的起点
        [s_start,t_start] = CalcSTCoordinate(row_start,col_start,s_list,t_list);
        s_dot_start = dp_st_s_dot(row_start,col_start);
    end
    cur_s_dot = (s_end - s_start) / (t_end - t_start);
    cur_s_dot2 = (cur_s_dot - s_dot_start)/(t_end - t_start);
    % 计算推荐速度代价
    cost_ref_speed = w_cost_ref_speed * (cur_s_dot - reference_speed)^2;
    % 计算加速度代价，这里注意，加速度不能超过车辆动力学上下限
    if cur_s_dot2 < 4 && cur_s_dot2 > -6
        cost_accel = w_cost_accel * cur_s_dot2^2;
    else
        % 超过车辆动力学限制，代价会增大很多倍
        cost_accel = 100000 * w_cost_accel * cur_s_dot2^2;
    end
    cost_obs = CalcObsCost(s_start,t_start,s_end,t_end,obs_st_s_in_set,obs_st_s_out_set,obs_st_t_in_set,obs_st_t_out_set,w_cost_obs);
    cost = cost_obs + cost_accel + cost_ref_speed;
end

function obs_cost = CalcObsCost(s_start,t_start,s_end,t_end,obs_st_s_in_set,obs_st_s_out_set,obs_st_t_in_set,obs_st_t_out_set,w_cost_obs)
% 该函数将计算边的障碍物代价
% 输入：边的起点终点s_start,t_start,s_end,t_end
%       障碍物信息 obs_st_s_in_set,obs_st_s_out_set,obs_st_t_in_set,obs_st_t_out_set
%       障碍物代价权重w_cost_obs
% 输出：边的障碍物代价obs_cost
  % 输出初始化
  obs_cost = 0;
  % 采样点的个数
  n = 5;
  % 采样时间间隔
  dt = (t_end - t_start)/(n - 1);
  % 边的斜率
  k = (s_end - s_start)/(t_end - t_start);
  for i = 1:n
      % 计算采样点的坐标
      t = t_start + (i - 1) * dt;
      s = s_start + k * (i - 1) * dt;
      % 遍历所有障碍物
      for j = 1:length(obs_st_s_in_set)
          if isnan(obs_st_s_in_set(j))
              continue;
          end
          % 计算点到st线段的最短距离
          vector1 = [obs_st_s_in_set(j);obs_st_t_in_set(j)] - [s;t];
          vector2 = [obs_st_s_out_set(j);obs_st_t_out_set(j)] - [s;t];
          vector3 = vector2 - vector1;
          min_dis = 0;
          dis1 = sqrt(vector1'*vector1);
          dis2 = sqrt(vector2'*vector2);
          dis3 = abs(vector1(1)*vector3(2) - vector1(2)*vector3(1))/sqrt(vector3'*vector3);
          if (vector1'*vector3 > 0 && vector2'*vector3 > 0) || (vector1'*vector3 < 0 && vector2'*vector3 < 0)
              min_dis = min(dis1,dis2);
          else
              min_dis = dis3;
          end
          obs_cost = obs_cost + CalcCollisionCost(w_cost_obs,min_dis); 
      end
  end
      
end

function collision_cost = CalcCollisionCost(w_cost_obs,min_dis)
  if abs(min_dis) < 0.5
      collision_cost = w_cost_obs;
  elseif abs(min_dis) > 0.5 && abs(min_dis) < 1.5
      % min_dis = 0.5    collision_cost = w_cost_obs^1;
      % min_dis = 1.5    collision_cost = w_cost_obs^0 = 1
      collision_cost = w_cost_obs^((0.5 - min_dis) + 1);
  else
      collision_cost = 0;
  end
end

function [s_value,t_value] = CalcSTCoordinate(row,col,s_list,t_list)
% 该函数将计算矩阵节点的s t 坐标
% 输入 row col 节点在矩阵的行号和列号
%      s_list t_list 采样间隔表
% 输出：s_value t_value 节点的 s t坐标
% 矩阵的(1,1) 代表的是最左上角的元素 s 最大 t 最小
% * 。。。。。。。。
% * 。。。。。。。。
% * 。。。。。。。。
% * 。。。。。。。。
% *****************

% 首先取出矩阵的行数
m = length(s_list);
% 1 1 对应的是 s 的最大值 t 的最小值
s_value = s_list(m - row + 1);
t_value = t_list(col);
end

== matlab function testemplanner_cs_old/Audi_A8_Sedan_1/decision&planning module/EM Planner/stitch trajectory1 ==
  data: trajectory_x input; trajectory_x_final output; trajectory_y input; trajectory_heading input; trajectory_kappa input; trajectory_speed input; trajectory_accel input; trajectory_time input; stitch_x input; stitch_y input; stitch_heading input; stitch_kappa input; stitch_speed input; stitch_accel input; stitch_time input; trajectory_y_final output; trajectory_heading_final output; trajectory_kappa_final output; trajectory_speed_final output; trajectory_accel_final output; trajectory_time_final output
function [trajectory_x_final,trajectory_y_final,trajectory_heading_final,trajectory_kappa_final,...
          trajectory_speed_final,trajectory_accel_final,trajectory_time_final] = fcn(trajectory_x,...
          trajectory_y,trajectory_heading,trajectory_kappa,trajectory_speed,trajectory_accel,trajectory_time,...
          stitch_x,stitch_y,stitch_heading,stitch_kappa,stitch_speed,stitch_accel,stitch_time)
% 轨迹拼接，把stitch trajectory 拼到规划完成的轨迹上
n = 401 + 20;
trajectory_x_final = zeros(n,1);
trajectory_y_final = zeros(n,1);
trajectory_heading_final = zeros(n,1);
trajectory_kappa_final = zeros(n,1);
trajectory_speed_final = zeros(n,1);
trajectory_accel_final = zeros(n,1);
trajectory_time_final = zeros(n,1);

trajectory_x_final = [stitch_x;trajectory_x];
trajectory_y_final = [stitch_y;trajectory_y];
trajectory_heading_final = [stitch_heading;trajectory_heading];
trajectory_kappa_final = [stitch_kappa;trajectory_kappa];
trajectory_speed_final = [stitch_speed;trajectory_speed];
trajectory_accel_final = [stitch_accel;trajectory_accel];
trajectory_time_final = [stitch_time;trajectory_time];

== matlab function testemplanner_cs_old/Audi_A8_Sedan_1/decision&planning module/referenceline provider/MATLAB Function10 ==
  data: referenceline_x_init input; referenceline_x output; referenceline_y_init input; w_cost_smooth input; w_cost_length input; w_cost_ref input; x_lb input; x_ub input; y_lb input; y_ub input; referenceline_y output
function [referenceline_x,referenceline_y] = ...
    fcn(referenceline_x_init,referenceline_y_init,w_cost_smooth,w_cost_length,w_cost_ref,x_lb,x_ub,y_lb,y_ub)
%该函数将平滑referenceline
%使用二次规划
%0.5x'Hx + f'x = min
% lb < x < ub
% 输入 referenceline x,y,init未平滑的参考线
% w_cost_smooth,w_cost_length,w_cost_ref 平滑代价，紧凑代价，几何相似代价权重系数
% x_lb,x_ub,y_lb,y_ub 允许x,y变化的上下界
% 输出 referenceline_x,referenceline_y 平滑后的参考线

%在这里为了简化，不使用参考线拼接算法
%计算量问题通过调度解决，规划周期为100ms，只要在100ms计算完就可以
%如果到最后计算速度成问题在优化，目前暂时不使用拼接

%simulink无法直接使用自带的二次规划函数，需要从外部引入

coder.extrinsic("quadprog");
% 二次规划形式
% H1 = w_cost_smooth*(A1'*A1) + w_cost_length*(A2'*A2) + w_cost_ref*(A3'*A3)
% f = -2 * w_cost_ref * referenceline_init
% x'H1x + f'x = 0.5 * x'(2H1)*x + f'x
% A1 = [1  0 -2  0  1  0
%       0  1  0 -2  0  1
%             1  0 -2  0  1  0
%             0  1  0 -2  0  1
%                   ...............
%A2 = [1  0 -1  0
%      0  1  0 -1
%            1  0 -1  0
%            0  1  0 -1
%                  ...........
%A3 为单位矩阵
%设置求解矩阵规模，因为参考线初始点一共181个，每个点有两个坐标，所以求解矩阵规模是362个
n = 181;
%referenceline初始化
referenceline_x = zeros(n,1);
referenceline_y = zeros(n,1);

A1 = zeros(2 * n - 4, 2 * n);
A2 = zeros(2 * n - 2, 2 * n);
A3 = eye(2 * n, 2 * n);
f = zeros(2 * n, 1);
lb = zeros(2 * n, 1);
ub = zeros(2 * n, 1);
persistent is_first_run;
persistent pre_result_x;
persistent pre_result_y;
persistent pre_referenceline_x_init;
persistent pre_referenceline_y_init;

if isempty(is_first_run)
    is_first_run = 0;
    for i = 1 : n
        f(2 * i - 1) = referenceline_x_init(i);
        f(2 * i) = referenceline_y_init(i);
        lb(2 * i - 1) = f(2 * i - 1) + x_lb;
        ub(2 * i - 1) = f(2 * i - 1) + x_ub;
        lb(2 * i) = f(2 * i) + y_lb;
        ub(2 * i) = f(2 * i) + y_ub;
    end

    for j = 1 :2: 2 * n - 5
        A1(j , j) = 1;
        A1(j , j + 2) = -2;
        A1(j , j + 4) = 1;
        A1(j + 1, j + 1) = 1;
        A1(j + 1, j + 3) = -2;
        A1(j + 1, j + 5) = 1;
    end

    for k = 1 : 2: 2 * n - 3
        A2(k, k) = 1;
        A2(k, k + 2) = -1;
        A2(k + 1, k + 1) = 1;
        A2(k + 1, k + 3) = -1;
    end

    H1 = w_cost_smooth * (A1'*A1) + w_cost_length * (A2'*A2) + w_cost_ref * A3;
    H = 2 * H1;
    %用 referenceline 的初值作为二次规划的迭代起点
    X0 = f;
    f = -2 * w_cost_ref * f;
    %二次规划求解
    X = quadprog(H,f,[],[],[],[],lb,ub,X0);
    %将结果输出到referenceline中
    for i = 1 : n
        referenceline_x(i) = X(2 * i - 1);
        referenceline_y(i) = X(2 * i);
    end
    pre_result_x = referenceline_x;
    pre_result_y = referenceline_y;
    pre_referenceline_x_init = referenceline_x_init;
    pre_referenceline_y_init = referenceline_y_init;
else
    if pre_referenceline_x_init(1) == referenceline_x_init(1) && ...
            pre_referenceline_y_init(1) == referenceline_y_init(1)
        %起点相同，可以认为本周期和上周期的referenceline_init 一模一样，就直接复用上个周期的结果
        referenceline_x = pre_result_x;
        referenceline_y = pre_result_y;
    else
        %起点不同。重复第一次运行的逻辑
        for i = 1 : n
            f(2 * i - 1) = referenceline_x_init(i);
            f(2 * i) = referenceline_y_init(i);
            lb(2 * i - 1) = f(2 * i - 1) + x_lb;
            ub(2 * i - 1) = f(2 * i - 1) + x_ub;
            lb(2 * i) = f(2 * i) + y_lb;
            ub(2 * i) = f(2 * i) + y_ub;
        end

        for j = 1 : 2: 2 * n - 5
            A1(i , i) = 1;
            A1(i , i + 2) = -2;
            A1(i , i + 4) = 1;
            A1(i + 1, i + 1) = 1;
            A1(i + 1, i + 3) = -2;
            A1(i + 1, i + 5) = 1;
        end

        for k = 1 : 2: 2 * n - 3
            A2(i, i) = 1;
            A2(i, i + 2) = -1;
            A2(i + 1, i + 1) = 1;
            A2(i + 1, i + 3) = -1;
        end

        H1 = w_cost_smooth * (A1'*A1) + w_cost_length * (A2'*A2) + w_cost_ref * A3;
        H = 2 * H1;
        %用 referenceline 的初值作为二次规划的迭代起点
        X0 = f;
        f = -2 * w_cost_ref * f;
        %二次规划求解
        X = quadprog(H,f,[],[],[],[],lb,ub,X0);
        %将结果输出到referenceline中
        for i = 1 : n
            referenceline_x(i) = X(2 * i - 1);
            referenceline_y(i) = X(2 * i);
        end
        pre_result_x = referenceline_x;
        pre_result_y = referenceline_y;
        pre_referenceline_x_init = referenceline_x_init;
        pre_referenceline_y_init = referenceline_y_init;
        
    end
    
end

== matlab function testemplanner_cs_old/Audi_A8_Sedan_2/PathFollower_Preview_1/LateralController/Calculate delta steering error/eml_delta_steering_error ==
  data: v_x_vehicle input; v_x_vehicle_Min input; t_Preview_LatCtrl input; delta_steeringwheeltotal output; v_y_vehicle input; yawrate_vehicle input; CorneringStiffness_Tyres_Front input; CorneringStiffness_Tyres_Rear input; m_vehicle_total input; inertia_z_vehicle_total input; e_Lat input size=10; Pos_x_CoG_Vehicle input; wheelbase input; RefreshCounter parameter
function delta_steeringwheeltotal = eml_delta_steering_error(v_x_vehicle,v_x_vehicle_Min,t_Preview_LatCtrl,v_y_vehicle,yawrate_vehicle,CorneringStiffness_Tyres_Front,CorneringStiffness_Tyres_Rear,m_vehicle_total,inertia_z_vehicle_total,e_Lat,Pos_x_CoG_Vehicle,wheelbase,RefreshCounter)

delta_steeringwheeltotal = emlfcn_delta_steering_error(v_x_vehicle,v_x_vehicle_Min,t_Preview_LatCtrl,v_y_vehicle,yawrate_vehicle,CorneringStiffness_Tyres_Front,CorneringStiffness_Tyres_Rear,m_vehicle_total,inertia_z_vehicle_total,e_Lat,Pos_x_CoG_Vehicle,wheelbase,RefreshCounter);

% end function
